simulink model "main"  (R2022a)
settings: Solver=VariableStepAuto  StartTime=0.0  StopTime=50  RelTol=1e-3
undefined symbols (not defined in the file or in its folder): xc7z007sclg400
libraries: hdlBasic x73, vmcUtilities x1
settings Model: Creator=viktor  LastModifiedBy=viktor

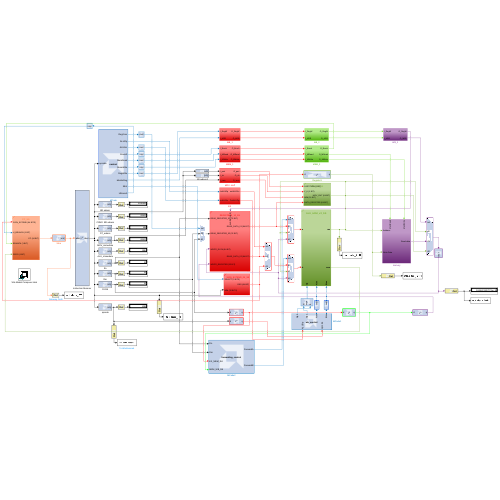
[thumbnail: Simulink's stored preview of the top-level diagram]
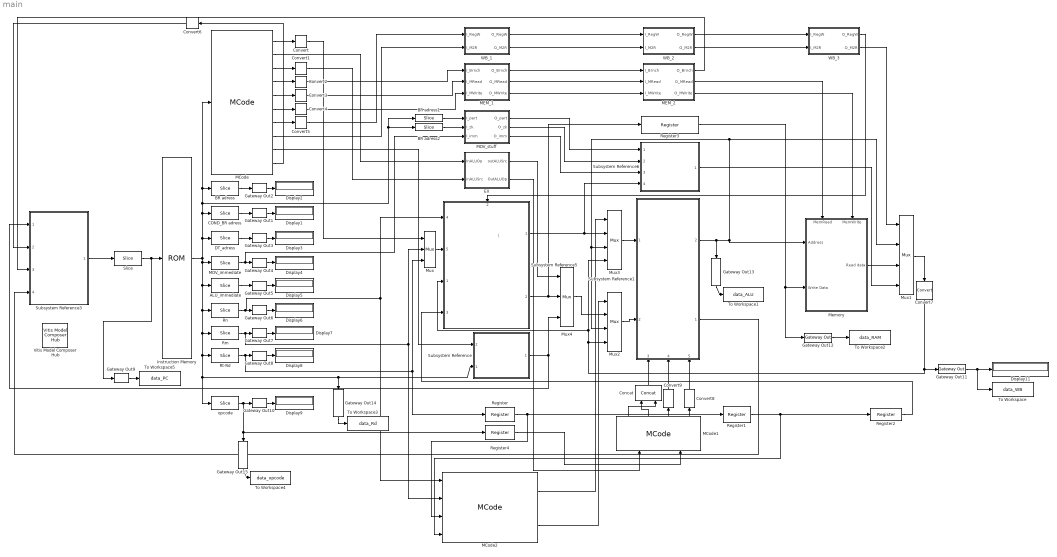
== system main ==
  note: (
  ALU_immediate : hdlBasic/Slice  nbits=1  boolean_output=off  mode=Two Bit Locations  bit1=21  base1=LSB of Input  bit0=10  base0=LSB of Input  XmcBlockStatus=1  maskContainerNames=group1  block_type=slice  block_config=sysgen:Slice_config
  BR adress : hdlBasic/Slice  nbits=1  boolean_output=off  mode=Two Bit Locations  bit1=25  base1=LSB of Input  bit0=0  base0=LSB of Input  XmcBlockStatus=1  maskContainerNames=group1  block_type=slice  block_config=sysgen:Slice_config
  BR adress1 : hdlBasic/Slice  nbits=1  boolean_output=off  mode=Two Bit Locations  bit1=23  base1=LSB of Input  bit0=22  base0=LSB of Input  XmcBlockStatus=1  maskContainerNames=group1  block_type=slice  block_config=sysgen:Slice_config
  BR adress2 : hdlBasic/Slice  nbits=1  boolean_output=off  mode=Two Bit Locations  bit1=24  base1=LSB of Input  bit0=24  base0=LSB of Input  XmcBlockStatus=1  maskContainerNames=group1  block_type=slice  block_config=sysgen:Slice_config
  COND_BR adress : hdlBasic/Slice  nbits=1  boolean_output=off  mode=Two Bit Locations  bit1=23  base1=LSB of Input  bit0=5  base0=LSB of Input  XmcBlockStatus=1  maskContainerNames=group1  block_type=slice  block_config=sysgen:Slice_config
  Concat : hdlBasic/Concat  num_inputs=2  XmcBlockStatus=1  maskContainerNames=group1  block_type=concat  block_config=sysgen:Concat_config
  Convert{,1..6} (7 alike) : hdlBasic/Convert  gui_display_data_type=Boolean  arith_type=Boolean  n_bits=16  bin_pt=14  float_type=Single  exp_bits=8  fraction_bits=24  quantization=Truncate  overflow=Wrap  en=off  latency=0  pipeline=off  XmcBlockStatus=1  maskContainerNames=group2  block_type=convert  block_config=sysgen:Convert_config  block_width=595  block_height=885
  Convert7 : hdlBasic/Convert  gui_display_data_type=Fixed-point  arith_type=Unsigned  n_bits=64  bin_pt=0  float_type=Single  exp_bits=8  fraction_bits=24  quantization=Truncate  overflow=Wrap  en=off  latency=0  pipeline=off  XmcBlockStatus=1  maskContainerNames=group2  block_type=convert  block_config=sysgen:Convert_config  block_width=595  block_height=885
  Convert8 : hdlBasic/Convert  gui_display_data_type=Fixed-point  arith_type=Unsigned  n_bits=1  bin_pt=0  float_type=Single  exp_bits=8  fraction_bits=24  quantization=Truncate  overflow=Wrap  en=off  latency=0  pipeline=off  XmcBlockStatus=1  maskContainerNames=group2  block_type=convert  block_config=sysgen:Convert_config  block_width=595  block_height=885
  Convert9 : hdlBasic/Convert  gui_display_data_type=Fixed-point  arith_type=Unsigned  n_bits=1  bin_pt=0  float_type=Single  exp_bits=8  fraction_bits=24  quantization=Truncate  overflow=Wrap  en=off  latency=0  pipeline=off  XmcBlockStatus=1  maskContainerNames=group2  block_type=convert  block_config=sysgen:Convert_config  block_width=595  block_height=885
  DT_adress : hdlBasic/Slice  nbits=1  boolean_output=off  mode=Two Bit Locations  bit1=20  base1=LSB of Input  bit0=12  base0=LSB of Input  XmcBlockStatus=1  maskContainerNames=group1  block_type=slice  block_config=sysgen:Slice_config
  Display{1..9,11} (10 alike) : Display
  EX : Subsystem
  Gateway Out{1..15} (15 alike) : hdlBasic/Gateway Out  inherit_from_input=off  hdl_port=on  rows=1  columns=1  UseAsDAC=off  DACChannel='1'  interface=None  automatic_assignment=on  address_offset=hex2dec('00')  intf_name=''  intf_description=''  timing_constraint=None  locs_specified=off  LOCs={}  io_standard={}  XmcBlockStatus=1  maskContainerNames=group4  block_type=gatewayout  block_config=sysgen:gateway_out_config  block_width_w=590  block_height_w=620  block_width=620  block_height=750
  Instruction Memory : hdlBasic/ROM  depth=256  initVector=[2684354601, 2684354602, 2288714091, 2684354881, 2684354562, 2684354563, 3019899169, 2282357035, 2415919433, 2415919466, 2281832548, 4160749706, 2415920194, 2432697377, 402653174, 2283734015, 2283734015, 2283734015]  distributed_mem=Block RAM  rst=off  init_reg=0  en=off  latency=1  gui_display_data_type=Fixed-point  arith_type=Unsigned  n_bits=32  bin_pt=0  preci_type=Single  exp_width=8  frac_width=24  optimize=Area  use_rpm=on  simulation_type=fast_sim  XmcBlockStatus=1  maskContainerNames=tabcontainer1  block_type=sprom  block_config=sysgen:SPROM_config
  MCode : hdlBasic/MCode  mfname=control  explicit_period=off  period=0  iptable={ 'opcode', '' }  optable={ 'Reg2Loc', 'off'; 'ALUOp', 'off'; 'ALUSrc', 'off'; 'Branch', 'off'; 'MemRead', 'off'; 'MemWrite', 'off'; 'RegWrite', 'off'; 'MemtoReg', 'off'; 'SExt', 'off'; 'UBranch', 'off' }  enable_stdout=off  enable_debug=off  suppress_output='on'  defparams={}  hide_port_list={}  block_type=mcode  block_width=444  block_height=788
      settings: infoedit=Pass input values to a MATLAB function for evaluation in Xilinx fixed-point type. The input ports of the block are input arguments of the function. The output ports of the block are output arguments of the function.
  MCode1 : hdlBasic/MCode  mfname=alu_control  explicit_period=off  period=1  iptable={ 'ALUOp', ''; 'opcode', '' }  optable={ 'Op0', 'off'; 'Op1', 'off'; 'Ainv', 'off'; 'Binv', 'off' }  enable_stdout=off  enable_debug=off  suppress_output='on'  defparams={}  hide_port_list={}  block_type=mcode  block_width=444  block_height=788
      settings: infoedit=Pass input values to a MATLAB function for evaluation in Xilinx fixed-point type. The input ports of the block are input arguments of the function. The output ports of the block are output arguments of the function.
  MCode2 : hdlBasic/MCode  mfname=forwarding_control  explicit_period=off  period=1  iptable={ 'Rn', ''; 'Rm', ''; 'EX_MEM_Rd', ''; 'MEM_WB_Rd', '' }  optable={ 'ForwardA', 'off'; 'ForwardB', 'off' }  enable_stdout=off  enable_debug=off  suppress_output='on'  defparams={}  hide_port_list={}  block_type=mcode  block_width=444  block_height=788
      settings: infoedit=Pass input values to a MATLAB function for evaluation in Xilinx fixed-point type. The input ports of the block are input arguments of the function. The output ports of the block are output arguments of the function.
  MEM_1 : Subsystem
  MEM_2 : Subsystem
  MOV_immediate : hdlBasic/Slice  nbits=1  boolean_output=off  mode=Two Bit Locations  bit1=20  base1=LSB of Input  bit0=5  base0=LSB of Input  XmcBlockStatus=1  maskContainerNames=group1  block_type=slice  block_config=sysgen:Slice_config
  MOV_stuff : Subsystem
  Memory : Subsystem
      settings: PortSchema="{\"entries\":[{\"content\":{\"sides\":[{\"content\":{\"connectorIds\":[\"In1\",\"In2\"]},\"type\":\"ConnectorPlacement.EquallySpacedRectSide\",\"uuid\":\"fc822c90-6391-42bc-910b-8255d660ef87\"},{\"content\":{\"connectorIds\":[\"Out1\"],\"side\":\"RIGHT\"},\"type\":\"ConnectorPlacement.EquallySpacedRectSide\",\"uuid\":\"b7dafd51-688c-4f54-93d2-8b60bc11f8cc\"},{\"content\":{\"connectorIds\":[\"In3\",\"In4\"],\"side\":\"TOP\"},\"type\":\"ConnectorPlacement.EquallySpacedRectSide\",\"uuid\":\"0f6376c4-5bf8-45a1-ac1c-0c59da9315eb\"}]},\"type\":\"ConnectorPlacement.EquallySpacedConnector\",\"uuid\":\"b340d8d8-eca0-4644-8498-1e3882a6bb1d\"}],\"packageUris\":[\"http://schema.mathworks.com/mf0/Connector/R2020b\"],\"version\":\"1.0\"}"
  Mux : hdlBasic/Mux  inputs=2  en=off  latency=0  precision=User Defined  arith_type=Unsigned  n_bits=5  bin_pt=0  quantization=Truncate  overflow=Wrap  XmcBlockStatus=1  maskContainerNames=tabcontainer1  block_type=mux  block_config=sysgen:Mux_config
  Mux1 : hdlBasic/Mux  inputs=3  en=off  latency=0  precision=User Defined  arith_type="Signed  (2's comp)"  n_bits=64  bin_pt=0  quantization=Truncate  overflow=Wrap  XmcBlockStatus=1  maskContainerNames=tabcontainer1  block_type=mux  block_config=sysgen:Mux_config
  Mux2 : hdlBasic/Mux  inputs=3  en=off  latency=0  precision=User Defined  arith_type=Unsigned  n_bits=64  bin_pt=0  quantization=Truncate  overflow=Wrap  XmcBlockStatus=1  maskContainerNames=tabcontainer1  block_type=mux  block_config=sysgen:Mux_config
  Mux3 : hdlBasic/Mux  inputs=3  en=off  latency=0  precision=User Defined  arith_type=Unsigned  n_bits=64  bin_pt=0  quantization=Truncate  overflow=Wrap  XmcBlockStatus=1  maskContainerNames=tabcontainer1  block_type=mux  block_config=sysgen:Mux_config
  Mux4 : hdlBasic/Mux  inputs=2  en=off  latency=0  precision=User Defined  arith_type=Unsigned  n_bits=64  bin_pt=0  quantization=Truncate  overflow=Wrap  XmcBlockStatus=1  maskContainerNames=tabcontainer1  block_type=mux  block_config=sysgen:Mux_config
  Register{,1..4} (5 alike) : hdlBasic/Register  init=0  rst=off  en=off  XmcBlockStatus=1  maskContainerNames=tabcontainer1  block_type=register  block_config=sysgen:Register_config
  Rm : hdlBasic/Slice  nbits=1  boolean_output=off  mode=Two Bit Locations  bit1=20  base1=LSB of Input  bit0=16  base0=LSB of Input  XmcBlockStatus=1  maskContainerNames=group1  block_type=slice  block_config=sysgen:Slice_config
  Rn : hdlBasic/Slice  nbits=1  boolean_output=off  mode=Two Bit Locations  bit1=9  base1=LSB of Input  bit0=5  base0=LSB of Input  XmcBlockStatus=1  maskContainerNames=group1  block_type=slice  block_config=sysgen:Slice_config
  Rt-Rd : hdlBasic/Slice  nbits=1  boolean_output=off  mode=Two Bit Locations  bit1=4  base1=LSB of Input  bit0=0  base0=LSB of Input  XmcBlockStatus=1  maskContainerNames=group1  block_type=slice  block_config=sysgen:Slice_config
  Slice : hdlBasic/Slice  nbits=1  boolean_output=off  mode=Two Bit Locations  bit1=7  base1=LSB of Input  bit0=0  base0=LSB of Input  XmcBlockStatus=1  maskContainerNames=group1  block_type=slice  block_config=sysgen:Slice_config
  Subsystem Reference : Subsystem  ReferencedSubsystem=SIGN_EXTEND_04_SS
      settings: PortSchema="{\"entries\":[{\"content\":{\"sides\":[{\"content\":{\"connectorIds\":[\"In2\",\"In1\"]},\"type\":\"ConnectorPlacement.EquallySpacedRectSide\",\"uuid\":\"1f917b85-6c19-4021-b508-0322bc161091\"},{\"content\":{\"connectorIds\":[\"Out1\"],\"side\":\"RIGHT\"},\"type\":\"ConnectorPlacement.EquallySpacedRectSide\",\"uuid\":\"93679915-3f6f-4b2e-9d4c-059131291ae8\"},{\"content\":{\"connectorIds\":[],\"side\":\"TOP\"},\"type\":\"ConnectorPlacement.EquallySpacedRectSide\",\"uuid\":\"c93e9737-35e1-4627-9222-28c2580f8718\"}]},\"type\":\"ConnectorPlacement.EquallySpacedConnector\",\"uuid\":\"ef19b6d7-2fc9-4582-b1fd-e7eb48768cf3\"}],\"packageUris\":[\"http://schema.mathworks.com/mf0/Connector/R2020b\"],\"version\":\"1.0\"}"
  Subsystem Reference1 : Subsystem  ReferencedSubsystem=ALU_64bit_v2_SS
      settings: PortSchema="{\"entries\":[{\"content\":{\"sides\":[{\"content\":{\"connectorIds\":[\"In1\",\"In2\"]},\"type\":\"ConnectorPlacement.EquallySpacedRectSide\",\"uuid\":\"b0a3a7a9-36fe-4986-a920-8e1e0821803a\"},{\"content\":{\"connectorIds\":[\"Out2\",\"Out1\"],\"side\":\"RIGHT\"},\"type\":\"ConnectorPlacement.EquallySpacedRectSide\",\"uuid\":\"10c339d2-e840-4e02-85ac-6788d5737be6\"},{\"content\":{\"connectorIds\":[],\"side\":\"TOP\"},\"type\":\"ConnectorPlacement.EquallySpacedRectSide\",\"uuid\":\"4daec9fe-3b0b-40d8-8161-2d842ccbf554\"},{\"content\":{\"connectorIds\":[\"In3\",\"In4\",\"In5\"],\"side\":\"BOTTOM\"},\"type\":\"ConnectorPlacement.EquallySpacedRectSide\",\"uuid\":\"478afad8-1ed0-4536-a1b3-c75edbd94cd4\"}]},\"type\":\"ConnectorPlacement.EquallySpacedConnector\",\"uuid\":\"666e4614-10b0-492b-8518-540098145fb8\"}],\"packageUris\":[\"http://schema.mathworks.com/mf0/Connector/R2020b\"],\"version\":\"1.0\"}"
  Subsystem Reference3 : Subsystem  ReferencedSubsystem=PC_SS
  Subsystem Reference5 : Subsystem  ReferencedSubsystem=REGISTERS_10_SS
      settings: PortSchema="{\"entries\":[{\"content\":{\"sides\":[{\"content\":{\"connectorIds\":[\"In4\",\"In5\",\"In1\",\"In3\"]},\"type\":\"ConnectorPlacement.EquallySpacedRectSide\",\"uuid\":\"b0a3a7a9-36fe-4986-a920-8e1e0821803a\"},{\"content\":{\"connectorIds\":[\"Out1\",\"Out2\"],\"side\":\"RIGHT\"},\"type\":\"ConnectorPlacement.EquallySpacedRectSide\",\"uuid\":\"10c339d2-e840-4e02-85ac-6788d5737be6\"},{\"content\":{\"connectorIds\":[\"In2\"],\"side\":\"TOP\"},\"type\":\"ConnectorPlacement.EquallySpacedRectSide\",\"uuid\":\"4daec9fe-3b0b-40d8-8161-2d842ccbf554\"}]},\"type\":\"ConnectorPlacement.EquallySpacedConnector\",\"uuid\":\"666e4614-10b0-492b-8518-540098145fb8\"}],\"packageUris\":[\"http://schema.mathworks.com/mf0/Connector/R2020b\"],\"version\":\"1.0\"}"
  Subsystem Reference6 : Subsystem  ReferencedSubsystem=MOV_05_SS
  To Workspace : ToWorkspace  VariableName=data_WB  SaveFormat=Timeseries  SampleTime=-1
  To Workspace1 : ToWorkspace  VariableName=data_ALU  SaveFormat=Timeseries  SampleTime=-1
  To Workspace2 : ToWorkspace  VariableName=data_RAM  SaveFormat=Timeseries  SampleTime=-1
  To Workspace3 : ToWorkspace  VariableName=data_Rd  SaveFormat=Timeseries  SampleTime=-1
  To Workspace4 : ToWorkspace  VariableName=data_opcode  SaveFormat=Timeseries  SampleTime=-1
  To Workspace5 : ToWorkspace  VariableName=data_PC  SaveFormat=Timeseries  SampleTime=-1
  Vitis Model Composer Hub : vmcUtilities/Vitis Model Composer Hub  Tag=genX  CodeGeneration=off  TargetDirectory=./code  ExportType=AI Engines  IpVendor=xilinx.com  IpLibrary=hls  IpVersion=1.0  IpHWLanguage=Verilog  AieCompilerOptions={}  AieSimulatorOptions={}  CreateTestbench=off  TestbenchStackSize=10  RunAieSim=off  AieSimTimeout=50000  RunAieSimProfiling=off  LaunchVitisAnalyzer=off  PlotOutput=off  RunX86Sim=off  X86SimTimeout=10  GenHwImage=off  PlatformType=Not Specified  HwSystemType=Baremetal  HwValidationTarget=hw  ProjDevice=xc7z007sclg400-1  ProjDevicePart=xc7z007sclg400-1  SamplePeriod=-1  ClockFrequency=200  DataPathParallelism=1  xilinxfamily=zynq  part=xc7z007s  speed=-1  package=clg400  directory=./netlist  testbench=off  incr_netlist=off  synthesis_tool=Vivado  clock_wrapper=Clock Enables  dbl_ovrd=According to Block Masks  dcm_input_clock_period=10  sysclk_period=10  simulink_period=1  eval_field=0  LogFileName=''  NThreads=4
  WB_1 : Subsystem
  WB_2 : Subsystem
  WB_3 : Subsystem
  opcode : hdlBasic/Slice  nbits=1  boolean_output=off  mode=Two Bit Locations  bit1=31  base1=LSB of Input  bit0=21  base0=LSB of Input  XmcBlockStatus=1  maskContainerNames=group1  block_type=slice  block_config=sysgen:Slice_config
  wires:
  Rt-Rd/1 -> Gateway Out8/1, Register/1, Mux/3
  opcode/1 -> Gateway Out15/1, Register4/1, Gateway Out10/1
  BR adress/1 -> Gateway Out2/1
  Gateway Out2/1 -> Display2/1
  Rn/1 -> Subsystem Reference5/4, MCode2/1, Gateway Out6/1
  Rm/1 -> Gateway Out7/1, MCode2/2, Mux/2
  ALU_immediate/1 -> Gateway Out5/1
  Instruction Memory/1 -> opcode/1, Gateway Out14/1, Subsystem Reference/1, Rt-Rd/1, Rm/1, Rn/1, ALU_immediate/1, MOV_immediate/1, BR adress1/1, BR adress2/1, MCode/1, BR adress/1, COND_BR adress/1, DT_adress/1
  MOV_immediate/1 -> Gateway Out4/1, MOV_stuff/3(I_imm)
  Subsystem Reference5/2 -> Register3/1, Mux4/2
  MCode/1 -> Convert/1
  Mux1/1 -> Convert7/1
  Memory/1(Read data) -> Mux1/3
  Subsystem Reference1/2 -> Mux3/3, Mux2/3, Mux1/2, Memory/1(Address), Gateway Out13/1
  Mux2/1 -> Subsystem Reference1/2
  MCode1/2 -> Concat/1
  MCode1/1 -> Concat/2
  Concat/1 -> Subsystem Reference1/3
  Mux3/1 -> Subsystem Reference1/1
  Subsystem Reference5/1 -> Subsystem Reference6/4, Mux3/2
  Register1/1 -> Register2/1, MCode2/4
  Register/1 -> MCode2/3, Register1/1
  Register2/1 -> Subsystem Reference5/3
  MCode2/1 -> Mux3/1
  MCode2/2 -> Mux2/1
  Mux4/1 -> Mux2/2
  Subsystem Reference/1 -> Mux4/3, Subsystem Reference3/1
  MCode/9 -> Subsystem Reference/2
  Subsystem Reference3/1 -> Slice/1
  Slice/1 -> Gateway Out9/1, Instruction Memory/1
  MCode/3 -> Convert1/1
  MCode/2 -> EX/1(InALUOp)
  EX/2(OutALUOp) -> MCode1/1
  EX/1(outALUSrc) -> Mux4/1
  MEM_1/2(O_MRead) -> MEM_2/2(I_MRead)
  MEM_1/1(O_Brnch) -> MEM_2/1(I_Brnch)
  MEM_2/2(O_MRead) -> Memory/3(MemRead)
  MEM_2/3(O_MWrite) -> Memory/4(MemWrite)
  MEM_2/1(O_Brnch) -> Subsystem Reference3/3
  WB_1/2(O_M2R) -> WB_2/2(I_M2R)
  WB_1/1(O_RegW) -> WB_2/1(I_RegW)
  WB_2/2(O_M2R) -> WB_3/2(I_M2R)
  WB_2/1(O_RegW) -> WB_3/1(I_RegW)
  WB_3/2(O_M2R) -> Mux1/1
  WB_3/1(O_RegW) -> Subsystem Reference5/2
  Subsystem Reference6/1 -> Mux1/4
  MEM_1/3(O_MWrite) -> MEM_2/3(I_MWrite)
  MOV_stuff/3(O_imm) -> Subsystem Reference6/3
  MOV_stuff/2(O_zk) -> Subsystem Reference6/2
  MOV_stuff/1(O_part) -> Subsystem Reference6/1
  BR adress2/1 -> MOV_stuff/2(I_zk)
  BR adress1/1 -> MOV_stuff/1(I_part)
  Gateway Out1/1 -> Display1/1
  COND_BR adress/1 -> Gateway Out1/1
  Gateway Out3/1 -> Display3/1
  DT_adress/1 -> Gateway Out3/1
  Gateway Out4/1 -> Display4/1
  Gateway Out5/1 -> Display5/1
  Gateway Out6/1 -> Display6/1
  Gateway Out7/1 -> Display7/1
  MCode/10 -> Convert6/1
  MCode/8 -> WB_1/2(I_M2R)
  MCode/4 -> Convert2/1
  MCode/7 -> Convert5/1
  MCode/5 -> Convert3/1
  MCode/6 -> Convert4/1
  Gateway Out11/1 -> To Workspace/1, Display11/1
  Mux/1 -> Subsystem Reference5/5
  Gateway Out10/1 -> Display9/1
  Gateway Out8/1 -> Display8/1
  Convert/1 -> Mux/1
  Convert1/1 -> EX/2(inALUSrc)
  Convert2/1 -> MEM_1/1(I_Brnch)
  Convert3/1 -> MEM_1/2(I_MRead)
  Convert4/1 -> MEM_1/3(I_MWrite)
  Convert5/1 -> WB_1/1(I_RegW)
  Convert6/1 -> Subsystem Reference3/2
  Convert7/1 -> Subsystem Reference5/1, Mux3/4, Mux2/4, Gateway Out11/1
  Subsystem Reference1/1 -> Subsystem Reference3/4
  MCode1/3 -> Convert9/1
  MCode1/4 -> Convert8/1
  Convert8/1 -> Subsystem Reference1/5
  Convert9/1 -> Subsystem Reference1/4
  Gateway Out9/1 -> To Workspace5/1
  Gateway Out12/1 -> To Workspace2/1
  Gateway Out13/1 -> To Workspace1/1
  Register3/1 -> Gateway Out12/1, Memory/2(Write Data)
  Register4/1 -> MCode1/2
  Gateway Out14/1 -> To Workspace3/1
  Gateway Out15/1 -> To Workspace4/1

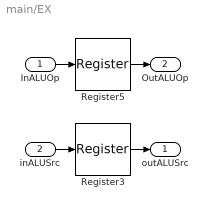
== system main/EX ==
  InALUOp : Inport
  inALUSrc : Inport  Port=2
  Register3 : hdlBasic/Register  init=0  rst=off  en=off  XmcBlockStatus=1  maskContainerNames=tabcontainer1  block_type=register  block_config=sysgen:Register_config
  Register5 : hdlBasic/Register  init=0  rst=off  en=off  XmcBlockStatus=1  maskContainerNames=tabcontainer1  block_type=register  block_config=sysgen:Register_config
  outALUSrc : Outport
  OutALUOp : Outport  Port=2
  wires:
  inALUSrc/1 -> Register3/1
  Register3/1 -> outALUSrc/1
  InALUOp/1 -> Register5/1
  Register5/1 -> OutALUOp/1

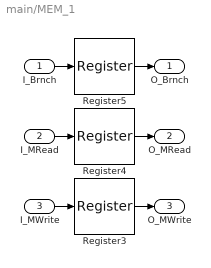
== system main/MEM_1 ==
  I_Brnch : Inport
  I_MRead : Inport  Port=2
  I_MWrite : Inport  Port=3
  Register3 : hdlBasic/Register  init=0  rst=off  en=off  XmcBlockStatus=1  maskContainerNames=tabcontainer1  block_type=register  block_config=sysgen:Register_config
  Register4 : hdlBasic/Register  init=0  rst=off  en=off  XmcBlockStatus=1  maskContainerNames=tabcontainer1  block_type=register  block_config=sysgen:Register_config
  Register5 : hdlBasic/Register  init=0  rst=off  en=off  XmcBlockStatus=1  maskContainerNames=tabcontainer1  block_type=register  block_config=sysgen:Register_config
  O_Brnch : Outport
  O_MRead : Outport  Port=2
  O_MWrite : Outport  Port=3
  wires:
  Register3/1 -> O_MWrite/1
  Register5/1 -> O_Brnch/1
  I_Brnch/1 -> Register5/1
  I_MRead/1 -> Register4/1
  Register4/1 -> O_MRead/1
  I_MWrite/1 -> Register3/1

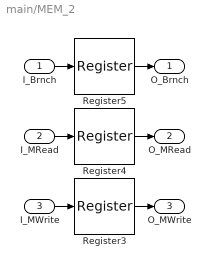
== system main/MEM_2 ==
  I_Brnch : Inport
  I_MRead : Inport  Port=2
  I_MWrite : Inport  Port=3
  Register3 : hdlBasic/Register  init=0  rst=off  en=off  XmcBlockStatus=1  maskContainerNames=tabcontainer1  block_type=register  block_config=sysgen:Register_config
  Register4 : hdlBasic/Register  init=0  rst=off  en=off  XmcBlockStatus=1  maskContainerNames=tabcontainer1  block_type=register  block_config=sysgen:Register_config
  Register5 : hdlBasic/Register  init=0  rst=off  en=off  XmcBlockStatus=1  maskContainerNames=tabcontainer1  block_type=register  block_config=sysgen:Register_config
  O_Brnch : Outport
  O_MRead : Outport  Port=2
  O_MWrite : Outport  Port=3
  wires:
  Register3/1 -> O_MWrite/1
  Register5/1 -> O_Brnch/1
  I_Brnch/1 -> Register5/1
  I_MRead/1 -> Register4/1
  Register4/1 -> O_MRead/1
  I_MWrite/1 -> Register3/1

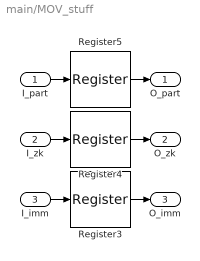
== system main/MOV_stuff ==
  I_part : Inport
  I_zk : Inport  Port=2
  I_imm : Inport  Port=3
  Register3 : hdlBasic/Register  init=0  rst=off  en=off  XmcBlockStatus=1  maskContainerNames=tabcontainer1  block_type=register  block_config=sysgen:Register_config
  Register4 : hdlBasic/Register  init=0  rst=off  en=off  XmcBlockStatus=1  maskContainerNames=tabcontainer1  block_type=register  block_config=sysgen:Register_config
  Register5 : hdlBasic/Register  init=0  rst=off  en=off  XmcBlockStatus=1  maskContainerNames=tabcontainer1  block_type=register  block_config=sysgen:Register_config
  O_part : Outport
  O_zk : Outport  Port=2
  O_imm : Outport  Port=3
  wires:
  Register4/1 -> O_zk/1
  I_imm/1 -> Register3/1
  Register5/1 -> O_part/1
  Register3/1 -> O_imm/1
  I_part/1 -> Register5/1
  I_zk/1 -> Register4/1

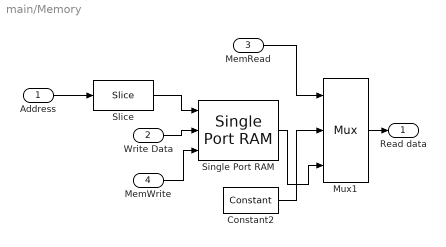
== system main/Memory ==
  Address : Inport
  Write Data : Inport  Port=2
  MemRead : Inport  Port=3
  MemWrite : Inport  Port=4
  Constant2 : hdlBasic/Constant  const=0  gui_display_data_type=Fixed-point  arith_type=Unsigned  n_bits=32  bin_pt=0  preci_type=Single  exp_width=8  frac_width=24  explicit_period=off  period=1  XmcBlockStatus=1  maskContainerNames=tabcontainer1  block_type=constant  block_config=sysgen:Constant_config
  Mux1 : hdlBasic/Mux  inputs=2  en=off  latency=0  precision=Full  arith_type=Unsigned  n_bits=16  bin_pt=14  quantization=Truncate  overflow=Wrap  XmcBlockStatus=1  maskContainerNames=tabcontainer1  block_type=mux  block_config=sysgen:Mux_config
  Single Port RAM : hdlBasic/Single Port RAM  depth=256  initVector=sin(pi*(0:15)/16)  distributed_mem=Block RAM  write_mode=Read After Write  rst=off  init_reg=0  en=off  optimize_latency=off  latency=1  optimize=Area  dbl_ovrd=off  simulation_type=fast_sim  XmcBlockStatus=1  maskContainerNames=tabcontainer1  block_type=spram  block_config=sysgen:SPRAM_config
  Slice : hdlBasic/Slice  nbits=1  boolean_output=off  mode=Two Bit Locations  bit1=7  base1=LSB of Input  bit0=0  base0=LSB of Input  XmcBlockStatus=1  maskContainerNames=group1  block_type=slice  block_config=sysgen:Slice_config
  Read data : Outport
  wires:
  Constant2/1 -> Mux1/2
  Write Data/1 -> Single Port RAM/2
  Mux1/1 -> Read data/1
  Address/1 -> Slice/1
  MemWrite/1 -> Single Port RAM/3
  Single Port RAM/1 -> Mux1/3
  Slice/1 -> Single Port RAM/1
  MemRead/1 -> Mux1/1

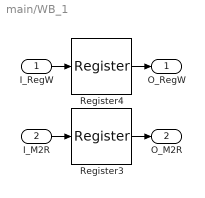
== system main/WB_1 ==
  I_RegW : Inport
  I_M2R : Inport  Port=2
  Register3 : hdlBasic/Register  init=0  rst=off  en=off  XmcBlockStatus=1  maskContainerNames=tabcontainer1  block_type=register  block_config=sysgen:Register_config
  Register4 : hdlBasic/Register  init=0  rst=off  en=off  XmcBlockStatus=1  maskContainerNames=tabcontainer1  block_type=register  block_config=sysgen:Register_config
  O_RegW : Outport
  O_M2R : Outport  Port=2
  wires:
  I_RegW/1 -> Register4/1
  Register3/1 -> O_M2R/1
  Register4/1 -> O_RegW/1
  I_M2R/1 -> Register3/1

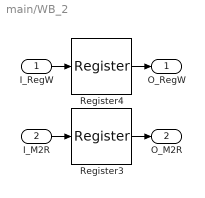
== system main/WB_2 ==
  I_RegW : Inport
  I_M2R : Inport  Port=2
  Register3 : hdlBasic/Register  init=0  rst=off  en=off  XmcBlockStatus=1  maskContainerNames=tabcontainer1  block_type=register  block_config=sysgen:Register_config
  Register4 : hdlBasic/Register  init=0  rst=off  en=off  XmcBlockStatus=1  maskContainerNames=tabcontainer1  block_type=register  block_config=sysgen:Register_config
  O_RegW : Outport
  O_M2R : Outport  Port=2
  wires:
  I_RegW/1 -> Register4/1
  Register3/1 -> O_M2R/1
  Register4/1 -> O_RegW/1
  I_M2R/1 -> Register3/1

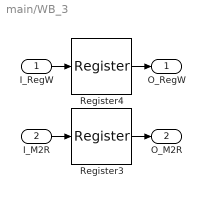
== system main/WB_3 ==
  I_RegW : Inport
  I_M2R : Inport  Port=2
  Register3 : hdlBasic/Register  init=0  rst=off  en=off  XmcBlockStatus=1  maskContainerNames=tabcontainer1  block_type=register  block_config=sysgen:Register_config
  Register4 : hdlBasic/Register  init=0  rst=off  en=off  XmcBlockStatus=1  maskContainerNames=tabcontainer1  block_type=register  block_config=sysgen:Register_config
  O_RegW : Outport
  O_M2R : Outport  Port=2
  wires:
  I_RegW/1 -> Register4/1
  Register3/1 -> O_M2R/1
  Register4/1 -> O_RegW/1
  I_M2R/1 -> Register3/1
